simulink model "FunctioncallSubsystem"  (R2015b)
settings: Solver=VariableStepAuto  StartTime=0.0  StopTime=10.0  RelTol=1e-3
settings Model: Creator=LUBO  LastModifiedBy=LUBO

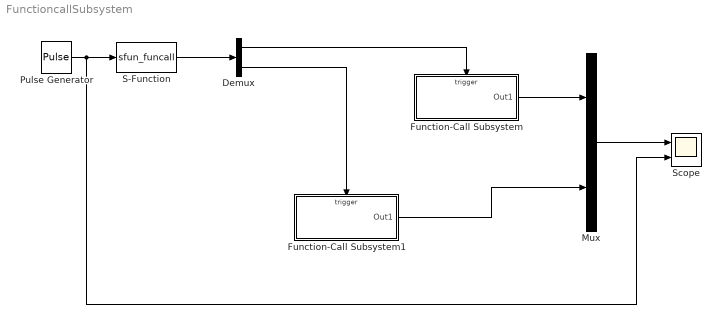
== system FunctioncallSubsystem ==
  Demux : Demux  Outputs=2
  Function-Call Subsystem : Subsystem  TreatAsAtomicUnit=on
  Function-Call Subsystem1 : Subsystem  TreatAsAtomicUnit=on
  Mux : Mux  Inputs=2
  Pulse Generator : DiscretePulseGenerator  PulseType=Time based  PulseWidth=50
  S-Function : S-Function  FunctionName=sfun_funcall  SFunctionDeploymentMode=off  EnableBusSupport=off
  Scope : Scope  NumInputPorts=2
  wires:
  Pulse Generator/1 -> Scope/2, S-Function/1
  S-Function/1 -> Demux/1
  Demux/2 -> Function-Call Subsystem1/Trigger
  Demux/1 -> Function-Call Subsystem/Trigger
  Function-Call Subsystem1/1(Out1) -> Mux/2
  Function-Call Subsystem/1(Out1) -> Mux/1
  Mux/1 -> Scope/1

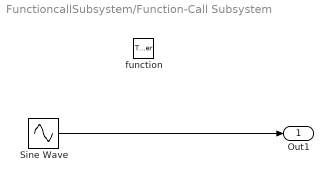
== system FunctioncallSubsystem/Function-Call Subsystem ==
  function : TriggerPort  TriggerType=function-call
  Sine Wave : Sin  SampleTime=0
  Out1 : Outport
  wires:
  Sine Wave/1 -> Out1/1

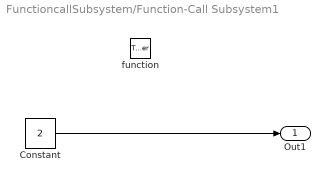
== system FunctioncallSubsystem/Function-Call Subsystem1 ==
  function : TriggerPort  TriggerType=function-call
  Constant : Constant  Value=2
  Out1 : Outport
  wires:
  Constant/1 -> Out1/1
